simulink model "gimbal_model_PID_131218"  (R2018b)
settings: Solver=FixedStepAuto  StartTime=0.0  StopTime=10  FixedStep=0.005  RelTol=1e-3
values from neighbouring files (symbols this model uses):
  DIM = data{4}    [gimbal_dynamics.m]
  DIS = data{5}    [gimbal_dynamics.m]
  I1 = data{1}    [gimbal_dynamics.m]    (also in macierze_inercji.m = sym('I1', [4 4]))
  I2 = data{2}    [gimbal_dynamics.m]    (also in macierze_inercji.m = sym('I2', [4 4]))
  I3 = data{3}    [gimbal_dynamics.m]    (also in macierze_inercji.m = sym('I3', [4 4]))
  M = [ud_ucz(3:p-1) ud_ucz(3:p-1).^2 ud_ucz(3:p-1).^3 ud_ucz(2:p-2) ud_ucz(2:p-2).^2 ud_ucz(2:p-2).^3 ud_ucz(1:p-3) ud_ucz(1:p-3).^2 ud_ucz(1:p-3).^3 yd_ucz(3:p-1) yd_ucz(3:p-1).^2 yd_ucz(3:p-1).^3 yd_ucz(2:p-2) yd_ucz(2:p-2).^2 yd_ucz(2:p-2).^3 yd_ucz(1:p-3) yd_ucz(1:p-3).^2 yd_ucz(1:p-3).^3]    [Identification_20191023.m]    (also in MI_beta.m = fillmissing(M,'spline'); gimbal_dynamics.m = data{6}; macierze_inercji.m = sym('M', [1 3]))
  m = [m1 m2 m3]    [dynamika_gimbala_symbolicznie.m]    (also in dynamika_gimbala_symbolicznie_20190706.m; dynamika_gimbala_symbolicznie_20190825.m)
libraries: simulink_extras x15, nesl_utility x7, sm_lib x6, simulink x1
settings Model: Creator=Paweł Tymiński  LastModifiedBy=Paweł Tymiński
settings SolverCC: ZeroCrossAlgorithm=Adaptive
settings DebuggingCC: IgnoredZcDiagnostic=none
settings SFSimCC: SimUseLocalCustomCode=off
settings RTWCC: RTWUseLocalCustomCode=off
settings CodeAppCC: StateflowObjectComments=on
settings SimscapeCC: SimscapeNormalizeSystem=off

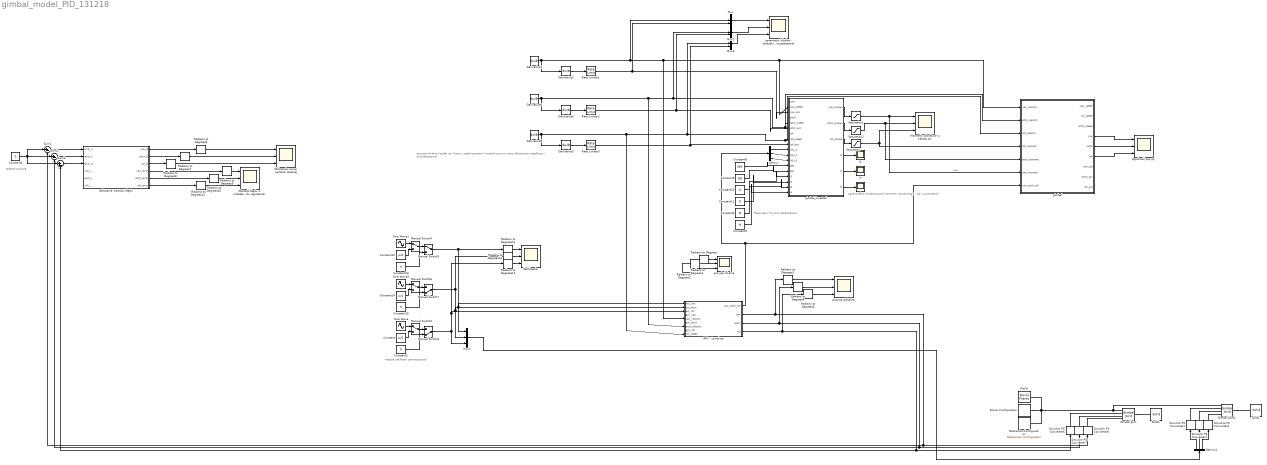
== system gimbal_model_PID_131218 ==
  note: zadana pozycja
  note: wejścia zakłóceń zewnętrznych
  note: pozycje lokalne każdej osi (wraz z ograniczeniami konstrukcyjnymi oraz obliczaniem prędkości i przyśpieszenia)
  note: Parametry fizyczne stabilizatora
  note: ograniczenia mechaniczne momentu obrotowego - do wyznaczenia
  Constant : Constant  Value=pi/2
  Constant10 : Constant  Value=I1
  Constant11 : Constant  Value=I2
  Constant12 : Constant  Value=pi/2
  Constant{2,6,13,15} (4 alike) : Constant  Value=0
  Constant14 : Constant  Value=pi/2
  Constant4 : Constant  Value=I3
  Constant5 : Constant  Value=M
  Constant8 : Constant  Value=DIM
  Constant9 : Constant  Value=DIS
  D : Scope
  Demux : Demux  Outputs=3
  Demux4 : Demux  Outputs=3
  Derivative{1..3,5..6,8} (6 alike) : Derivative
  G : Scope
  Gimbal Joint : sm_lib/Joints/Gimbal Joint  SenseConstraintForce=off  SenseConstraintForceX=off  SenseConstraintForceY=off  SenseConstraintForceZ=off  SenseConstraintTorque=off  SenseConstraintTorqueX=off  SenseConstraintTorqueY=off  SenseConstraintTorqueZ=off  SenseTotalForce=off  SenseTotalForceX=off  SenseTotalForceY=off  SenseTotalForceZ=off  SenseTotalTorque=off  SenseTotalTorqueX=off  SenseTotalTorqueY=off  SenseTotalTorqueZ=off  CompositeWrenchDir=FollowerOnBase  CompositeWrenchFrame=BaseFrame  RxEquilibriumPosition=0  RxEquilibriumPositionUnits=deg  RxSpringStiffness=0  RxSpringStiffnessUnits=N*m/deg  RxDampingCoefficient=0  RxDampingCoefficientUnits=N*m/(deg/s)  RxTorqueActuationMode=ComputedTorque  RxMotionActuationMode=InputMotion  RxSensePosition=off  RxSenseVelocity=off  RxSenseAcceleration=off  RxSenseTorqueForce=off  RxPositionTargetSpecify=off  RxPositionTargetPriority=High  RxPositionTargetValue=0  RxPositionTargetValueUnits=deg  RxVelocityTargetSpecify=off  RxVelocityTargetPriority=High  RxVelocityTargetValue=0  RxVelocityTargetValueUnits=deg/s  RyEquilibriumPosition=0  RyEquilibriumPositionUnits=deg  RySpringStiffness=0  RySpringStiffnessUnits=N*m/deg  RyDampingCoefficient=0  RyDampingCoefficientUnits=N*m/(deg/s)  RyTorqueActuationMode=ComputedTorque  RyMotionActuationMode=InputMotion  RySensePosition=off  RySenseVelocity=off  RySenseAcceleration=off  RySenseTorqueForce=off  RyPositionTargetSpecify=off  RyPositionTargetPriority=High  RyPositionTargetValue=0  RyPositionTargetValueUnits=deg  RyVelocityTargetSpecify=off  RyVelocityTargetPriority=High  RyVelocityTargetValue=0  RyVelocityTargetValueUnits=deg/s  RzEquilibriumPosition=0  RzEquilibriumPositionUnits=deg  RzSpringStiffness=0  RzSpringStiffnessUnits=N*m/deg  RzDampingCoefficient=0  RzDampingCoefficientUnits=N*m/(deg/s)  RzTorqueActuationMode=ComputedTorque  RzMotionActuationMode=InputMotion  RzSensePosition=off  RzSenseVelocity=off  RzSenseAcceleration=off  RzSenseTorqueForce=off  RzPositionTargetSpecify=off  RzPositionTargetPriority=High  RzPositionTargetValue=0  RzPositionTargetValueUnits=deg  RzVelocityTargetSpecify=off  RzVelocityTargetPriority=High  RzVelocityTargetValue=0  RzVelocityTargetValueUnits=deg/s
      settings: SourceProductName=Simscape Multibody
  Gimbal Joint1 : sm_lib/Joints/Gimbal Joint  SenseConstraintForce=off  SenseConstraintForceX=off  SenseConstraintForceY=off  SenseConstraintForceZ=off  SenseConstraintTorque=off  SenseConstraintTorqueX=off  SenseConstraintTorqueY=off  SenseConstraintTorqueZ=off  SenseTotalForce=off  SenseTotalForceX=off  SenseTotalForceY=off  SenseTotalForceZ=off  SenseTotalTorque=off  SenseTotalTorqueX=off  SenseTotalTorqueY=off  SenseTotalTorqueZ=off  CompositeWrenchDir=FollowerOnBase  CompositeWrenchFrame=BaseFrame  RxEquilibriumPosition=0  RxEquilibriumPositionUnits=deg  RxSpringStiffness=0  RxSpringStiffnessUnits=N*m/deg  RxDampingCoefficient=0  RxDampingCoefficientUnits=N*m/(deg/s)  RxTorqueActuationMode=ComputedTorque  RxMotionActuationMode=InputMotion  RxSensePosition=off  RxSenseVelocity=off  RxSenseAcceleration=off  RxSenseTorqueForce=off  RxPositionTargetSpecify=off  RxPositionTargetPriority=High  RxPositionTargetValue=0  RxPositionTargetValueUnits=deg  RxVelocityTargetSpecify=off  RxVelocityTargetPriority=High  RxVelocityTargetValue=0  RxVelocityTargetValueUnits=deg/s  RyEquilibriumPosition=0  RyEquilibriumPositionUnits=deg  RySpringStiffness=0  RySpringStiffnessUnits=N*m/deg  RyDampingCoefficient=0  RyDampingCoefficientUnits=N*m/(deg/s)  RyTorqueActuationMode=ComputedTorque  RyMotionActuationMode=InputMotion  RySensePosition=off  RySenseVelocity=off  RySenseAcceleration=off  RySenseTorqueForce=off  RyPositionTargetSpecify=off  RyPositionTargetPriority=High  RyPositionTargetValue=0  RyPositionTargetValueUnits=deg  RyVelocityTargetSpecify=off  RyVelocityTargetPriority=High  RyVelocityTargetValue=0  RyVelocityTargetValueUnits=deg/s  RzEquilibriumPosition=0  RzEquilibriumPositionUnits=deg  RzSpringStiffness=0  RzSpringStiffnessUnits=N*m/deg  RzDampingCoefficient=0  RzDampingCoefficientUnits=N*m/(deg/s)  RzTorqueActuationMode=ComputedTorque  RzMotionActuationMode=InputMotion  RzSensePosition=off  RzSenseVelocity=off  RzSenseAcceleration=off  RzSenseTorqueForce=off  RzPositionTargetSpecify=off  RzPositionTargetPriority=High  RzPositionTargetValue=0  RzPositionTargetValueUnits=deg  RzVelocityTargetSpecify=off  RzVelocityTargetPriority=High  RzVelocityTargetValue=0  RzVelocityTargetValueUnits=deg/s
      settings: SourceProductName=Simscape Multibody
  H : Scope
  IMU - żyroskop : Subsystem
  Manual Switch{2,4..6} (4 alike) : ManualSwitch
  Manual Switch3 : ManualSwitch  CurrentSetting=0
  Manual Switch7 : ManualSwitch  CurrentSetting=0
  MechanismConfiguration : sm_lib/Utilities/Mechanism Configuration  UniformGravity=Constant  GravityVector=[0 0 -9.80665]  GravityUnits=m/s^2  LinearizationDelta=0.001
  Momenty obrotowe w kazdej osi : Scope  NumInputPorts=3
  Mux{,1..3} (4 alike) : Mux  Inputs=3
  Obliczanie nowej wartości zadanej : Scope  NumInputPorts=3
  Obliczanie wartości błędu : MATLAB Function  TreatAsAtomicUnit=on
  Radians to Degrees{,1..14} (15 alike) : simulink_extras/Transformations/Radians to Degrees
  Rate Limiter1 : RateLimiter  RisingSlewLimit=10  FallingSlewLimit=-10  SampleTimeMode=inherited
  Rate Limiter2 : RateLimiter  RisingSlewLimit=10  FallingSlewLimit=-10  SampleTimeMode=inherited
  Rate Limiter3 : RateLimiter  RisingSlewLimit=10  FallingSlewLimit=-10  SampleTimeMode=inherited
  Saturation : Saturate  UpperLimit=10  LowerLimit=-10
  Saturation1 : Saturate  UpperLimit=10  LowerLimit=-10
  Saturation2 : Saturate  UpperLimit=10  LowerLimit=-10
  Simulink-PS Converter{1..3,6..8} (6 alike) : nesl_utility/Simulink-PS Converter  PhysicalDomain=network_engine_domain  SubClassName=ps_input  LeftPortType=input  RightPortType=output  PseudoPeriodic=off  Frequencies=[]  NoiseDistribution=none  NoiseParameters=[]  Unit=rad  AffineConversion=off  FilteringAndDerivatives=filter  SimscapeFilterOrder=2  InputFilterTimeConstant=0.001  UdotUserProvided=0
  Sine Wave : Sin  Amplitude=pi/16  Frequency=0.5  SampleTime=0
  Sine Wave1 : Sin  Amplitude=pi/16  Frequency=0.5  SampleTime=0
  Sine Wave2 : Sin  Amplitude=pi/16  Frequency=0.5  SampleTime=0
  Solid1 : sm_lib/Body Elements/Solid  InertiaType=Custom  Mass=0.01  MassUnits=kg  CenterOfMass=[10 30 21]  CenterOfMassUnits=mm  MomentsOfInertia=[1 1 1]  MomentsOfInertiaUnits=kg*m^2  ProductsOfInertia=[0 0 0]  ProductsOfInertiaUnits=kg*m^2  BasedOnType=Density  Density=1000  DensityUnits=kg/m^3  DoExposeReferenceFrame=on  SerializedFrames=<Frames/>  GraphicType=FromGeometry  MarkerShape=Sphere  MarkerSize=10  GraphicVisPropType=SimpleVisualProperties  GraphicDiffuseColor=[1.0 0.2 0.2]  GraphicSpecularColor=[0.5 0.5 0.5 1.0]  GraphicAmbientColor=[0.15 0.15 0.15 1.0]  GraphicEmissiveColor=[0.0 0.0 0.0 1.0]  GraphicShininess=75  GraphicOpacity=1.0  GeometryShape=Brick  RectangleSize=[1 1]  RectangleSizeUnits=m  BrickDimensions=[3 1 2]  BrickDimensionUnits=cm  CylinderRadius=1  CylinderRadiusUnits=m  CylinderLength=1  CylinderLengthUnits=m  SphereRadius=1  SphereRadiusUnits=m  EllipsoidRadii=[1 1 1]  EllipsoidRadiiUnits=m  ExtrusionCrossSection=[1 1; -1 1; -1 -1; 1 -1]  ExtrusionCrossSectionUnits=m  ExtrusionLength=1  ExtrusionLengthUnits=m  PolygonNumSides=3  PolygonOuterRadius=1  PolygonOuterRadiusUnits=m  ExtGeomFileType=STL  ExtGeomFileName=D:\OneDrive - Politechnika Warszawska\STUDIA\MGR\PRACA_MATERIALY\models\xiaomi-yi-action-cam-1.snapshot.2\YI ACTION CAM.STL  ExtGeomFileUnits=mm  RevolutionCrossSection=[1 1; 1 -1; 2 -1; 2 1]  RevolutionCrossSectionUnits=m  RevolutionExtent=Full  RevolutionAngle=180  RevolutionAngleUnits=deg
  Solid2 : sm_lib/Body Elements/Solid  InertiaType=Custom  Mass=0.01  MassUnits=kg  CenterOfMass=[10 30 21]  CenterOfMassUnits=mm  MomentsOfInertia=[1 1 1]  MomentsOfInertiaUnits=kg*m^2  ProductsOfInertia=[0 0 0]  ProductsOfInertiaUnits=kg*m^2  BasedOnType=Density  Density=1000  DensityUnits=kg/m^3  DoExposeReferenceFrame=on  SerializedFrames=<Frames/>  GraphicType=FromGeometry  MarkerShape=Sphere  MarkerSize=10  GraphicVisPropType=SimpleVisualProperties  GraphicDiffuseColor=[0.0 0.0 1.0]  GraphicSpecularColor=[0.5 0.5 0.5 1.0]  GraphicAmbientColor=[0.15 0.15 0.15 1.0]  GraphicEmissiveColor=[0.0 0.0 0.0 1.0]  GraphicShininess=75  GraphicOpacity=1.0  GeometryShape=Brick  RectangleSize=[1 1]  RectangleSizeUnits=m  BrickDimensions=[2 2 1]  BrickDimensionUnits=cm  CylinderRadius=1  CylinderRadiusUnits=m  CylinderLength=1  CylinderLengthUnits=m  SphereRadius=1  SphereRadiusUnits=m  EllipsoidRadii=[1 1 1]  EllipsoidRadiiUnits=m  ExtrusionCrossSection=[1 1; -1 1; -1 -1; 1 -1]  ExtrusionCrossSectionUnits=m  ExtrusionLength=1  ExtrusionLengthUnits=m  PolygonNumSides=3  PolygonOuterRadius=1  PolygonOuterRadiusUnits=m  ExtGeomFileType=STL  ExtGeomFileName=D:\OneDrive - Politechnika Warszawska\STUDIA\MGR\PRACA_MATERIALY\models\xiaomi-yi-action-cam-1.snapshot.2\YI ACTION CAM.STL  ExtGeomFileUnits=mm  RevolutionCrossSection=[1 1; 1 -1; 2 -1; 2 1]  RevolutionCrossSectionUnits=m  RevolutionExtent=Full  RevolutionAngle=180  RevolutionAngleUnits=deg
  Solver Configuration : nesl_utility/Solver Configuration  PhysicalDomain=network_engine_domain  SubClassName=solver  LeftPortType=input  RightPortType=generic  Tones=[]  Harmonics=[]  SimulateNoise=off  Profile=off  UseLocalSampling=off  EnableSwitchedLinearOptims=on  FrequencyDomain=off  UseCCode=off  RelTol=0.001  AbsTol=1e-06  MinStep=1e-09  ToWorkspace=off  RevertToSquareIcSolve=off  NumHomotopyIterations=100  PhasorMode=off  PhasorModeNumHarmonics=1  DoDC=off  ResidualTolerance=1e-09  UseLocalSolver=off  LocalSolverChoice=NE_BACKWARD_EULER_ADVANCER  LocalSolverSampleTime=0.001  DoFixedCost=off  MaxNonlinIter=3  MaxModeIter=2  LinearAlgebra=Sparse  EquationFormulation=NE_TIME_EF  DelaysMemoryBudget=1024  AutomaticFiltering=on  FilteringTimeConstant=0.001  PartitionStorageMethod=AS_NEEDED  PartitionMemoryBudget=1024
  Sum1 : Sum  Inputs=|+-
  Sum2 : Sum  Inputs=|+-
  Sum3 : Sum  Inputs=|+-
  Wartość błędu w układach lokalnych (do regulatora) : Scope  NumInputPorts=3
  World : sm_lib/Frames and Transforms/World Frame
  Zakłócenia : Scope  NumInputPorts=3
  Zgodność pozycji : Scope  NumInputPorts=3
  gimbal : Subsystem
  gimbal_inverted : MATLAB Function  TreatAsAtomicUnit=on
  "parametry lokalne - położenie, prędkość, przyśpieszenie" : Scope  NumInputPorts=3
  pozycja globalna : Scope  NumInputPorts=3
  pozycja lokalna : Scope  NumInputPorts=3
  wires:
  Constant6/1 -> Sum3/1, Sum2/1, Sum1/1
  Sine Wave/1 -> Manual Switch2/1
  Constant/1 -> Manual Switch2/2
  Manual Switch2/1 -> Manual Switch3/1
  Constant2/1 -> Manual Switch3/2
  Sum3/1 -> Obliczanie wartości błędu/3(error_3)
  Obliczanie wartości błędu/1(yaw_D) -> Radians to Degrees5/1
  Obliczanie wartości błędu/3(roll_D) -> Radians to Degrees8/1
  Obliczanie wartości błędu/2(pitch_D) -> Radians to Degrees7/1
  Sum1/1 -> Obliczanie wartości błędu/1(error_1)
  Sum2/1 -> Obliczanie wartości błędu/2(error_2)
  Radians to Degrees7/1 -> Obliczanie nowej wartości zadanej/2
  Radians to Degrees5/1 -> Obliczanie nowej wartości zadanej/1
  Radians to Degrees8/1 -> Obliczanie nowej wartości zadanej/3
  Radians to Degrees10/1 -> Wartość błędu w układach lokalnych (do regulatora)/2
  Radians to Degrees9/1 -> Wartość błędu w układach lokalnych (do regulatora)/1
  Obliczanie wartości błędu/4(yaw_error) -> Radians to Degrees9/1
  Radians to Degrees11/1 -> Wartość błędu w układach lokalnych (do regulatora)/3
  Obliczanie wartości błędu/6(roll_error) -> Radians to Degrees11/1
  Obliczanie wartości błędu/5(pitch_error) -> Radians to Degrees10/1
  Radians to Degrees12/1 -> Zakłócenia/1
  Radians to Degrees14/1 -> Zakłócenia/3
  Radians to Degrees13/1 -> Zakłócenia/2
  IMU - żyroskop/4(roll) -> Radians to Degrees6/1, Simulink-PS Converter6/1, Sum3/2
  IMU - żyroskop/2(yaw) -> Radians to Degrees3/1, Simulink-PS Converter8/1, Sum1/2
  IMU - żyroskop/3(pitch) -> Radians to Degrees4/1, Simulink-PS Converter7/1, Sum2/2
  Mux2/1 -> Demux4/1
  Demux4/1 -> Simulink-PS Converter1/1
  Demux4/2 -> Simulink-PS Converter2/1
  Demux4/3 -> Simulink-PS Converter3/1
  Constant8/1 -> gimbal_inverted/13(DIM)
  Constant9/1 -> gimbal_inverted/14(DIS)
  Constant10/1 -> gimbal_inverted/15(I1)
  Constant11/1 -> gimbal_inverted/16(I2)
  Constant4/1 -> gimbal_inverted/17(I3)
  Constant5/1 -> gimbal_inverted/18(M)
  IMU - żyroskop/1(yaw_pitch_roll) -> gimbal/7(yaw_pitch_roll), Demux/1
  Demux/2 -> gimbal_inverted/11(IMU_2)
  Demux/3 -> gimbal_inverted/12(IMU_3)
  Demux/1 -> gimbal_inverted/10(IMU_1)
  gimbal_inverted/2(pitch_torque) -> Saturation2/1
  gimbal_inverted/1(yaw_torque) -> Saturation1/1
  gimbal_inverted/3(roll_torque) -> Saturation/1
  Constant13/1 -> Manual Switch5/2
  Manual Switch4/1 -> Manual Switch5/1
  Constant12/1 -> Manual Switch4/2
  Sine Wave1/1 -> Manual Switch4/1
  Constant15/1 -> Manual Switch7/2
  Manual Switch6/1 -> Manual Switch7/1
  Constant14/1 -> Manual Switch6/2
  Sine Wave2/1 -> Manual Switch6/1
  Manual Switch5/1 -> Radians to Degrees12/1, Mux2/1, IMU - żyroskop/1(ext_yaw)
  Manual Switch7/1 -> Radians to Degrees13/1, IMU - żyroskop/2(ext_pitch), Mux2/2
  Manual Switch3/1 -> Mux2/3, IMU - żyroskop/3(ext_roll), Radians to Degrees14/1
  Derivative1/1 -> Derivative2/1, Mux/2, IMU - żyroskop/5(yaw_velocity), gimbal/1(yaw_velocity), gimbal_inverted/2(yaw_speed)
  Derivative5/1 -> Rate Limiter2/1
  Derivative3/1 -> Rate Limiter3/1
  Derivative6/1 -> Derivative5/1, IMU - żyroskop/7(pitch_velocity), Mux1/2, gimbal/2(pitch_velocity), gimbal_inverted/5(pitch_speed)
  Derivative8/1 -> Derivative3/1, IMU - żyroskop/9(roll_speed), Mux3/2, gimbal/3(roll_velocity), gimbal_inverted/8(roll_speed)
  gimbal/4(yaw) -> Zgodność pozycji/1
  gimbal/5(pitch) -> Zgodność pozycji/2
  gimbal/6(roll) -> Zgodność pozycji/3
  Saturation2/1 -> gimbal/5(pitch_moment), Momenty obrotowe w kazdej osi/2
  Saturation1/1 -> Momenty obrotowe w kazdej osi/1, gimbal/6(yaw_moment)  "yaw"
  Saturation/1 -> gimbal/4(roll_moment), Momenty obrotowe w kazdej osi/3
  Radians to Degrees2/1 -> pozycja lokalna/3
  Radians to Degrees1/1 -> pozycja lokalna/2
  Radians to Degrees/1 -> pozycja lokalna/1
  Radians to Degrees3/1 -> pozycja globalna/1
  Radians to Degrees4/1 -> pozycja globalna/2
  Radians to Degrees6/1 -> pozycja globalna/3
  ? -> Derivative1/1, Mux/1, Radians to Degrees/1, IMU - żyroskop/4(gim_yaw), Obliczanie wartości błędu/4(yaw_L), gimbal_inverted/1(yaw)
  ? -> Derivative6/1, IMU - żyroskop/6(gim_pitch), Radians to Degrees1/1, Obliczanie wartości błędu/5(pitch_L), Mux1/1, gimbal_inverted/4(pitch)
  ? -> IMU - żyroskop/8("gim_roll "), Radians to Degrees2/1, Obliczanie wartości błędu/6(roll_L), Mux3/1, gimbal_inverted/7(roll), Derivative8/1
  gimbal_inverted/4(D) -> D/1
  gimbal_inverted/5(H) -> H/1
  gimbal_inverted/6(G) -> G/1
  Mux/1 -> "parametry lokalne - położenie, prędkość, przyśpieszenie"/1
  Mux1/1 -> "parametry lokalne - położenie, prędkość, przyśpieszenie"/2
  Mux3/1 -> "parametry lokalne - położenie, prędkość, przyśpieszenie"/3
  Derivative2/1 -> Rate Limiter1/1
  Rate Limiter3/1 -> Mux3/3, gimbal_inverted/9(roll_acc)
  Rate Limiter2/1 -> Mux1/3, gimbal_inverted/6(pitch_acc)
  Rate Limiter1/1 -> Mux/3, gimbal_inverted/3(yaw_acc)
  connections:
  Simulink-PS Converter6/RConn1 -- Gimbal Joint/LConn2
  Simulink-PS Converter7/RConn1 -- Gimbal Joint/LConn3
  Gimbal Joint/RConn1 -- Solid1/RConn1
  World/RConn1 -- Gimbal Joint1/LConn1 -- Gimbal Joint/LConn1 -- MechanismConfiguration/RConn1 -- Solver Configuration/RConn1
  Simulink-PS Converter8/RConn1 -- Gimbal Joint/LConn4
  Simulink-PS Converter2/RConn1 -- Gimbal Joint1/LConn3
  Simulink-PS Converter1/RConn1 -- Gimbal Joint1/LConn2
  Simulink-PS Converter3/RConn1 -- Gimbal Joint1/LConn4
  Gimbal Joint1/RConn1 -- Solid2/RConn1

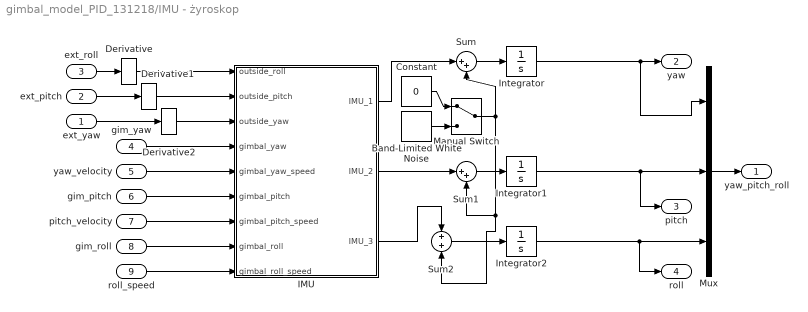
== system gimbal_model_PID_131218/IMU - żyroskop ==
  ext_yaw : Inport
  ext_pitch : Inport  Port=2
  ext_roll : Inport  Port=3
  gim_yaw : Inport  Port=4
  yaw_velocity : Inport  Port=5
  gim_pitch : Inport  Port=6
  pitch_velocity : Inport  Port=7
  "gim_roll " : Inport  Port=8
  roll_speed : Inport  Port=9
  Band-Limited White Noise : simulink/Sources/Band-Limited White Noise  Cov=[0.1]  Ts=0.1  seed=[23341]
  Constant : Constant  Value=0
  Derivative : Derivative
  Derivative1 : Derivative
  Derivative2 : Derivative
  IMU : MATLAB Function  TreatAsAtomicUnit=on
  Integrator : Integrator
  Integrator1 : Integrator
  Integrator2 : Integrator
  Manual Switch : ManualSwitch
  Mux : Mux  Inputs=3
  Sum : Sum  Inputs=|++
  Sum1 : Sum  Inputs=|++
  Sum2 : Sum
  yaw_pitch_roll : Outport
  yaw : Outport  Port=2
  pitch : Outport  Port=3
  roll : Outport  Port=4
  wires:
  roll_speed/1 -> IMU/9(gimbal_roll_speed)
  gim_pitch/1 -> IMU/6(gimbal_pitch)
  Mux/1 -> yaw_pitch_roll/1
  yaw_velocity/1 -> IMU/5(gimbal_yaw_speed)
  IMU/1(IMU_1) -> Sum/1
  pitch_velocity/1 -> IMU/7(gimbal_pitch_speed)
  ext_pitch/1 -> Derivative1/1
  ext_roll/1 -> Derivative/1
  ext_yaw/1 -> Derivative2/1
  "gim_roll "/1 -> IMU/8(gimbal_roll)
  gim_yaw/1 -> IMU/4(gimbal_yaw)
  IMU/3(IMU_3) -> Sum2/1
  IMU/2(IMU_2) -> Sum1/1
  Manual Switch/1 -> Sum2/2, Sum1/2, Sum/2
  Sum2/1 -> Integrator2/1
  Sum1/1 -> Integrator1/1
  Sum/1 -> Integrator/1
  Band-Limited White Noise/1 -> Manual Switch/2
  Constant/1 -> Manual Switch/1
  Derivative/1 -> IMU/1(outside_roll)
  Derivative1/1 -> IMU/2(outside_pitch)
  Derivative2/1 -> IMU/3(outside_yaw)
  Integrator/1 -> Mux/1, yaw/1
  Integrator2/1 -> roll/1, Mux/3
  Integrator1/1 -> pitch/1, Mux/2

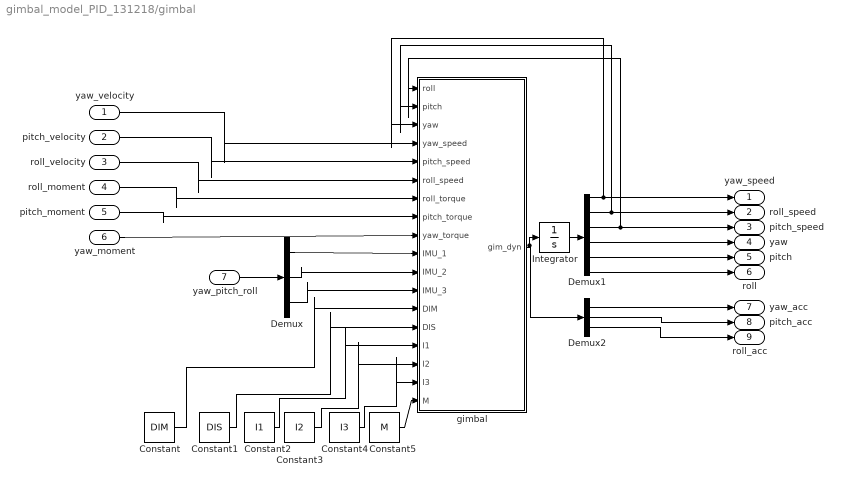
== system gimbal_model_PID_131218/gimbal ==
  yaw_velocity : Inport
  pitch_velocity : Inport  Port=2
  roll_velocity : Inport  Port=3
  roll_moment : Inport  Port=4
  pitch_moment : Inport  Port=5
  yaw_moment : Inport  Port=6
  yaw_pitch_roll : Inport  Port=7
  Constant : Constant  Value=DIM
  Constant1 : Constant  Value=DIS
  Constant2 : Constant  Value=I1
  Constant3 : Constant  Value=I2
  Constant4 : Constant  Value=I3
  Constant5 : Constant  Value=M
  Demux : Demux  Outputs=3
  Demux1 : Demux  Outputs=6
  Demux2 : Demux  Outputs=3
  Integrator : Integrator
  gimbal : MATLAB Function  TreatAsAtomicUnit=on
  yaw_speed : Outport
  roll_speed : Outport  Port=2
  pitch_speed : Outport  Port=3
  yaw : Outport  Port=4
  pitch : Outport  Port=5
  roll : Outport  Port=6
  yaw_acc : Outport  Port=7
  pitch_acc : Outport  Port=8
  roll_acc : Outport  Port=9
  wires:
  Demux/1 -> gimbal/10(IMU_1)
  Demux/3 -> gimbal/12(IMU_3)
  Demux/2 -> gimbal/11(IMU_2)
  gimbal/1(gim_dyn) -> Demux2/1, Integrator/1
  Demux1/2 -> roll_speed/1, gimbal/2(pitch)
  Demux1/1 -> yaw_speed/1, gimbal/3(yaw)
  yaw_pitch_roll/1 -> Demux/1
  pitch_velocity/1 -> gimbal/5(pitch_speed)
  roll_velocity/1 -> gimbal/6(roll_speed)
  roll_moment/1 -> gimbal/7(roll_torque)
  yaw_velocity/1 -> gimbal/4(yaw_speed)
  yaw_moment/1 -> gimbal/9(yaw_torque)
  pitch_moment/1 -> gimbal/8(pitch_torque)
  Demux1/3 -> pitch_speed/1, gimbal/1(roll)
  Integrator/1 -> Demux1/1
  Demux1/6 -> roll/1
  Demux1/5 -> pitch/1
  Demux1/4 -> yaw/1
  Constant5/1 -> gimbal/18(M)
  Constant4/1 -> gimbal/17(I3)
  Constant3/1 -> gimbal/16(I2)
  Constant2/1 -> gimbal/15(I1)
  Constant1/1 -> gimbal/14(DIS)
  Constant/1 -> gimbal/13(DIM)
  Demux2/1 -> yaw_acc/1
  Demux2/2 -> pitch_acc/1
  Demux2/3 -> roll_acc/1

== matlab function gimbal_model_PID_131218/IMU - żyroskop/IMU ==
  data: outside_roll input; IMU_1 output; outside_pitch input; outside_yaw input; gimbal_yaw input; gimbal_yaw_speed input; gimbal_pitch input; gimbal_pitch_speed input; gimbal_roll input; gimbal_roll_speed input; IMU_2 output; IMU_3 output

function [IMU_1, IMU_2, IMU_3] = IMU(outside_roll,outside_pitch,outside_yaw,gimbal_yaw ,gimbal_yaw_speed, gimbal_pitch ,gimbal_pitch_speed , gimbal_roll , gimbal_roll_speed  )
% kąty gimbala
theta_1 = gimbal_yaw ;
theta_2 = gimbal_pitch ;
theta_3 = gimbal_roll ;

J_0 =[1 0 0;
    0 cos(theta_1) -sin(theta_1);
   -sin(theta_2) cos(theta_2)*sin(theta_1) cos(theta_1)*cos(theta_2)];
Phi_0 = [outside_yaw; outside_pitch; outside_roll];

Omega_phi = J_0*Phi_0;

Omega = [gimbal_yaw_speed; gimbal_pitch_speed; gimbal_roll_speed];

J = [cos(theta_2)*cos(theta_3) sin(theta_3) 0;
    cos(theta_2)*sin(theta_3) cos(theta_3) 0;
    -sin(theta_2) 0 1];
A=J*(Omega_phi + Omega);

IMU_1 = A(1); %yaw
IMU_2 = A(2); %pitch
IMU_3 = A(3); %roll

end

== matlab function gimbal_model_PID_131218/Obliczanie wartości błędu ==
  data: error_1 input; yaw_D output; error_2 input; error_3 input; pitch_D output; roll_D output; yaw_L input; pitch_L input; roll_L input; yaw_error output; pitch_error output; roll_error output
function [yaw_D,pitch_D,roll_D, yaw_error, pitch_error, roll_error] = fcn(error_1,error_2,error_3,yaw_L, pitch_L, roll_L)
E=[cos(error_1)*cos(error_3)-sin(error_1)*sin(error_2)*sin(error_3) -cos(error_2)*sin(error_1) cos(error_1)*sin(error_1)+cos(error_3)*sin(error_1)*sin(error_2);
cos(error_3)*sin(error_1)+cos(error_1)*sin(error_2)*sin(error_2) cos(error_1)*cos(error_2) sin(error_1)*sin(error_3)-cos(error_1)*cos(error_3)*sin(error_2);
-cos(error_2)*sin(error_3) sin(error_2) cos(error_2)*cos(error_3)];



r12 = E(1,2);
r22 = E(2,2);
r31 = E(3,1);
r32 = E(3,2);
r33 = E(3,3);
yaw_D=atan2(-r12,r22);
pitch_D=asin(r32);
roll_D=atan2(-r31,r33);
yaw_error=yaw_D-yaw_L;
pitch_error=pitch_D-pitch_L;
roll_error=roll_D-roll_L;
end

== matlab function gimbal_model_PID_131218/gimbal_inverted ==
  data: yaw input; yaw_speed input; yaw_acc input; pitch input; pitch_speed input; pitch_acc input; roll input; yaw_torque output; roll_speed input; roll_acc input; IMU_1 input; IMU_2 input; IMU_3 input; DIM input; DIS input; I1 input; I2 input; I3 input; M input; pitch_torque output; roll_torque output; D output; H output; G output
function [yaw_torque, pitch_torque, roll_torque , D, H, G]  = gimbal_dynamics(yaw,yaw_speed,yaw_acc,pitch,pitch_speed,pitch_acc,roll,roll_speed, roll_acc,IMU_1,IMU_2,IMU_3,DIM,DIS,I1,I2,I3,M)

%stała grawitacji
g = 9.81;


%-------------ZMIENNE--------------
% odczyty z IMU
alpha_1 = IMU_1;
alpha_2 = IMU_2;
alpha_3 = IMU_3;
IMU = [alpha_1; alpha_2; alpha_3];
%predkosci katowe osiagane przez gimbal
 om_1 = yaw_speed ;
 om_2 = pitch_speed ;
 om_3 = roll_speed ;
Omega = [om_1; om_2; om_3];
%kąty osiagane aktualnie przez gimbal
 theta_1 = yaw ;
 theta_2 = pitch ;
 theta_3 = roll ;
 THETA = [theta_1; theta_2; theta_3];
% przyśpieszenia kątowe w osiach gimbala
 ACC = [yaw_acc;pitch_acc;roll_acc];

%---------------FUNKCJE---------------------

H = calculate_H_matrix(THETA,Omega,I1,I2,I3,DIM);
D = calculate_D_matrix(THETA,I1,I2,I3,DIM);
G = calculate_G_matrix(IMU,THETA,DIM,g,M,DIS);
Q = D*ACC+H+G;
yaw_torque = Q(1);
pitch_torque = Q(2);
roll_torque = Q(3);

end

== matlab function gimbal_model_PID_131218/gimbal/gimbal ==
  data: roll input; gim_dyn output; pitch input; yaw input; yaw_speed input; pitch_speed input; roll_speed input; roll_torque input; pitch_torque input; yaw_torque input; IMU_1 input; IMU_2 input; IMU_3 input; DIM input; DIS input; I1 input; I2 input; I3 input; M input
function gim_dyn = gimbal_dynamics(roll,pitch,yaw,yaw_speed,pitch_speed,roll_speed,roll_torque,pitch_torque,yaw_torque,IMU_1,IMU_2,IMU_3,DIM,DIS,I1,I2,I3,M)

%stała grawitacji
g = 9.81;

%ładowanie macierzy dot. masy i bezwładności gimbala
% data=cell(1,6);
% data = calculate_I_matrix(0);
% I1=data{1};
% I2=data{2};
% I3=data{3};
% DIM=data{4};
% DIS=data{5};
% M=data{6};
%-------------ZMIENNE--------------
% odczyty z IMU
alpha_1 = IMU_1;
alpha_2 = IMU_2;
alpha_3 = IMU_3;
IMU = [alpha_1; alpha_2; alpha_3];

% momenty generowane przez silnik - zmienne sterujace
 T1 = yaw_torque ;
 T2 = pitch_torque ;
 T3 = roll_torque ;
%predkosci katowe osiagane przez gimbal
 om_1 = yaw_speed ;
 om_2 = pitch_speed ;
 om_3 = roll_speed ;
Omega = [om_1; om_2; om_3];
%kąty osiagane aktualnie przez gimbal
 theta_1 = yaw ;
 theta_2 = pitch ;
 theta_3 = roll ;
    THETA = [theta_1; theta_2; theta_3];

%---------------FUNKCJE---------------------

H = calculate_H_matrix(THETA,Omega,I1,I2,I3,DIM);
D = calculate_D_matrix(THETA,I1,I2,I3,DIM);
Q = calculate_Q_matrix(T1,T2,T3,Omega);
G = calculate_G_matrix(IMU,THETA,DIM,g,M,DIS);

gim_dyn = [inv(D)\(Q-H-G); Omega];
end
